simulink model "AC_motor_KDB_Roto_Day_Quan"  (R2019a)
settings: Solver=VariableStepAuto  StartTime=0.0  StopTime=10.0  RelTol=1e-3
libraries: powerlib x13
settings Model: Creator=Admin  LastModifiedBy=Admin

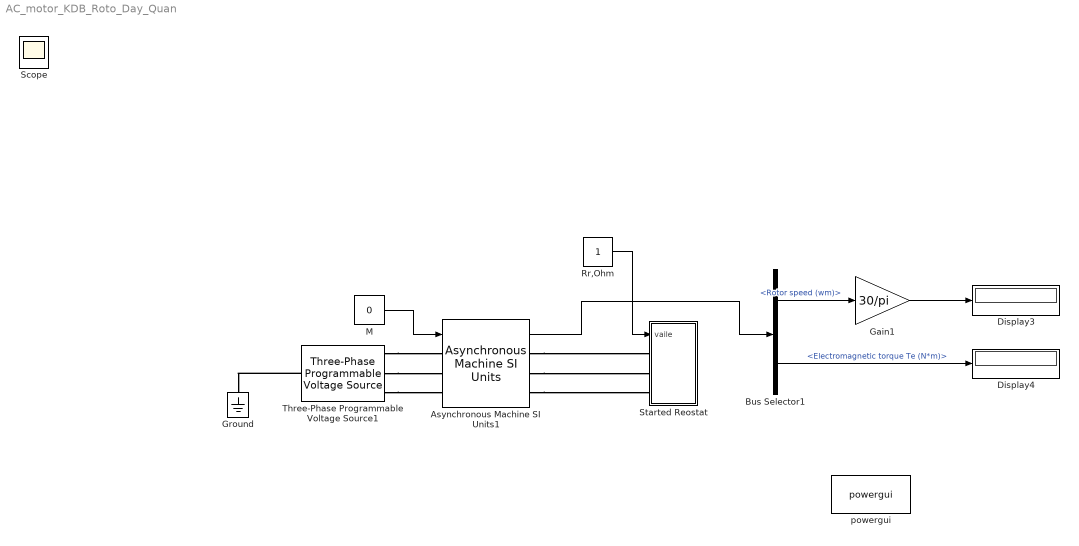
== system AC_motor_KDB_Roto_Day_Quan ==
  Asynchronous Machine SI Units1 : powerlib/Machines/Asynchronous Machine SI Units  RotorType=Wound  PresetModel="15:  5.4 HP (4KW)   400 V  50Hz 1430 RPM"  MechanicalLoad=Torque Tm  ShowDetailedParameters=on  ReferenceFrame=Stationary  Units=SI  MeasurementBus=off  NominalParameters=[1000 380 50]  Stator=[3.28 0.0039]  Rotor=[1.167 0.0039]  Cage1=[0.4155 0.002066]  Cage2=[0.4168 0.0003495]  Lm=0.1671  Mechanical="[0.0058  0 2]"  PolePairs=2  InitialConditions=[0 0 0 0 0 0 0 0]  SimulateSaturation=off  Saturation=[14.03593122, 27.81365428, 53.79336849, 72.68890987, 97.98006896, 148.6815601, 215.7428561, 302.9841135, 428.7778367 ; 230, 322, 414, 460, 506, 552, 598, 644, 690]  LoadFlowParameters=1492000  TsPowergui=0  TsBlock=-1  IterativeModel=Trapezoidal non iterative  IterativeDiscreteModel=Trapezoidal non iterative  Pmec=1.492e+006
      settings: SourceProductName=Simscape Electrical
  Bus Selector1 : BusSelector  OutputSignals=Mechanical.Rotor speed (wm),Mechanical.Electromagnetic torque Te (N*m)
  Display3 : Display
  Display4 : Display
  Gain1 : Gain  Gain=30/pi
  Ground : powerlib/Elements/Ground  LConnTagsString=a
      settings: SourceProductName=Simscape Electrical
  M : Constant  Value=0
  Rr,Ohm : Constant
  Scope : Scope
  Started Reostat : Subsystem
  Three-Phase Programmable Voltage Source1 : powerlib/Electrical Sources/Three-Phase Programmable Voltage Source  PositiveSequence="[380  0 50]"  VariationEntity=None  VariationType=Table of time-amplitude pairs  VariationTypeAlt=Step  VariationStep=0.5  VariationRate=10  VariationMagnitude=0.3  VariationFrequency=2  VariationTiming=[1 2]  VariationPhaseA=off  Amplitudes=[1 0.8 1.2 1.0]  TimeValues=[0 0.1 0.15 0.2]  HarmonicGeneration=off  HarmonicA=[3 0.2 -25 0]  HarmonicB=[2 0.15 35 2]  Timing="[0.05  3]"  BusType=swing  Pref=0  Qref=0  Qmin=-inf  Qmax=inf
      settings: SourceProductName=Simscape Electrical
  powergui : powerlib/powergui  Priority=1  SimulationMode=Continuous  SampleTime=50e-6  frequency=60  Iterations=50  frequencyindice=50  Pbase=100e6  ErrMax=1e-4  UnitsV=kV  UnitsW=MW  buscounter=0  FunctionMessages=off  echomessages=off  EnableUseOfTLC=off  CurrentSourceSwitches=off  DisableSnubberDevices=off  DisableRonSwitches=off  DisableVfSwitches=off  DisplayEquations=off  AutomaticDiscreteSolvers=off  SolverType=Tustin/Backward Euler (TBE)  Interpol=off  ExternalGateDelay=off  methode=off  Ts=100  x0status=blocks  SPID=on  SwTol=0  HookPort=off  NonlinearTolerance=0  nMaxIteration=15  ContinueOnMaxIteration=off  RestoreLinks=warning  ResistiveCurrentMeasurement=off  Frange=[0:2:500]  Ylog=off  Xlog=on  ShowGrid=off  save=off  variable=ZData  structure=0  ZoomFFT=off  StartTime=0.0  cycles=1  DisplayStyle=1  fundamental=60  FreqAxis=off  MaxFrequency=1000  frequencyindicesteady=1  RmsSteady=1  display=off
      settings: SourceProductName=Simscape Electrical
  wires:
  Asynchronous Machine SI Units1/1 -> Bus Selector1/1
  Bus Selector1/1 -> Gain1/1  "<Rotor speed (wm)>"
  Gain1/1 -> Display3/1
  Bus Selector1/2 -> Display4/1  "<Electromagnetic torque Te (N*m)>"
  M/1 -> Asynchronous Machine SI Units1/1
  Rr,Ohm/1 -> Started Reostat/1(vaile)
  connections:
  Three-Phase Programmable Voltage Source1/LConn1 -- Ground/LConn1
  Three-Phase Programmable Voltage Source1/RConn1 -- Asynchronous Machine SI Units1/LConn1
  Three-Phase Programmable Voltage Source1/RConn2 -- Asynchronous Machine SI Units1/LConn2
  Three-Phase Programmable Voltage Source1/RConn3 -- Asynchronous Machine SI Units1/LConn3
  Asynchronous Machine SI Units1/RConn3 -- Started Reostat/LConn3
  Asynchronous Machine SI Units1/RConn2 -- Started Reostat/LConn2
  Asynchronous Machine SI Units1/RConn1 -- Started Reostat/LConn1

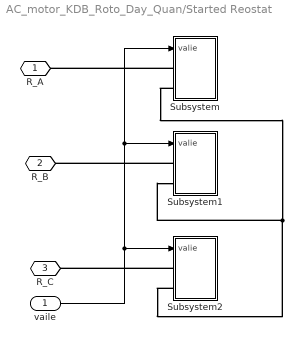
== system AC_motor_KDB_Roto_Day_Quan/Started Reostat ==
  vaile : Inport
  Subsystem : Subsystem
  Subsystem1 : Subsystem
  Subsystem2 : Subsystem
  R_A : PMIOPort  Side=Left
  R_B : PMIOPort  Port=2  Side=Left
  R_C : PMIOPort  Port=3  Side=Left
  wires:
  vaile/1 -> Subsystem2/1(valie), Subsystem1/1(valie), Subsystem/1(valie)
  connections:
  Subsystem/LConn1 -- R_A/RConn1
  Subsystem/LConn2 -- Subsystem2/LConn2 -- Subsystem1/LConn2
  Subsystem2/LConn1 -- R_C/RConn1
  Subsystem1/LConn1 -- R_B/RConn1

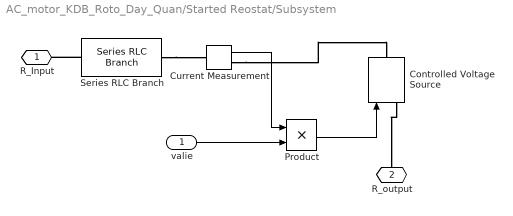
== system AC_motor_KDB_Roto_Day_Quan/Started Reostat/Subsystem ==
  valie : Inport
  Controlled Voltage Source : powerlib/Electrical Sources/Controlled Voltage Source  Initialize=on  Source_Type=AC  Amplitude=0  Phase=0  Frequency=0  Measurements=None
      settings: SourceProductName=Simscape Electrical
  Current Measurement : powerlib/Measurements/Current Measurement  PhasorSimulation=off  OutputType=Complex  PSBequivalent=0
      settings: SourceProductName=Simscape Electrical
  Product : Product
  Series RLC Branch : powerlib/Elements/Series RLC Branch  LConnTagsString=__new0  RConnTagsString=__new0  BranchType=R  Resistance=1  Inductance=1e-3  SetiL0=off  InitialCurrent=0  Capacitance=1e-6  Setx0=off  InitialVoltage=0  Measurements=None
      settings: SourceProductName=Simscape Electrical
  R_Input : PMIOPort  Side=Left
  R_output : PMIOPort  Port=2  Side=Left
  wires:
  Current Measurement/1 -> Product/1
  valie/1 -> Product/2
  Product/1 -> Controlled Voltage Source/1
  connections:
  Series RLC Branch/RConn1 -- Current Measurement/LConn1
  Current Measurement/RConn1 -- Controlled Voltage Source/RConn1
  Series RLC Branch/LConn1 -- R_Input/RConn1
  Controlled Voltage Source/LConn1 -- R_output/RConn1

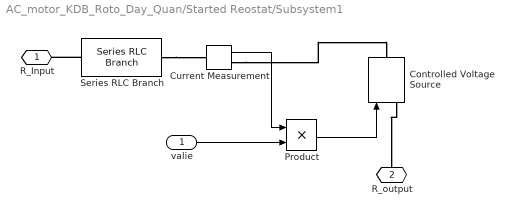
== system AC_motor_KDB_Roto_Day_Quan/Started Reostat/Subsystem1 ==
  valie : Inport
  Controlled Voltage Source : powerlib/Electrical Sources/Controlled Voltage Source  Initialize=on  Source_Type=AC  Amplitude=0  Phase=0  Frequency=0  Measurements=None
      settings: SourceProductName=Simscape Electrical
  Current Measurement : powerlib/Measurements/Current Measurement  PhasorSimulation=off  OutputType=Complex  PSBequivalent=0
      settings: SourceProductName=Simscape Electrical
  Product : Product
  Series RLC Branch : powerlib/Elements/Series RLC Branch  LConnTagsString=__new0  RConnTagsString=__new0  BranchType=R  Resistance=1  Inductance=1e-3  SetiL0=off  InitialCurrent=0  Capacitance=1e-6  Setx0=off  InitialVoltage=0  Measurements=None
      settings: SourceProductName=Simscape Electrical
  R_Input : PMIOPort  Side=Left
  R_output : PMIOPort  Port=2  Side=Left
  wires:
  Current Measurement/1 -> Product/1
  valie/1 -> Product/2
  Product/1 -> Controlled Voltage Source/1
  connections:
  Series RLC Branch/RConn1 -- Current Measurement/LConn1
  Current Measurement/RConn1 -- Controlled Voltage Source/RConn1
  Series RLC Branch/LConn1 -- R_Input/RConn1
  Controlled Voltage Source/LConn1 -- R_output/RConn1

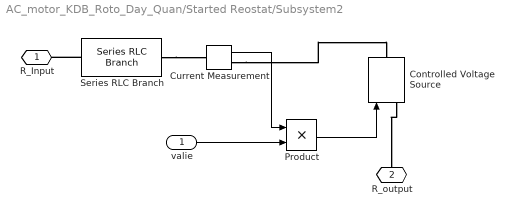
== system AC_motor_KDB_Roto_Day_Quan/Started Reostat/Subsystem2 ==
  valie : Inport
  Controlled Voltage Source : powerlib/Electrical Sources/Controlled Voltage Source  Initialize=on  Source_Type=AC  Amplitude=0  Phase=0  Frequency=0  Measurements=None
      settings: SourceProductName=Simscape Electrical
  Current Measurement : powerlib/Measurements/Current Measurement  PhasorSimulation=off  OutputType=Complex  PSBequivalent=0
      settings: SourceProductName=Simscape Electrical
  Product : Product
  Series RLC Branch : powerlib/Elements/Series RLC Branch  LConnTagsString=__new0  RConnTagsString=__new0  BranchType=R  Resistance=1  Inductance=1e-3  SetiL0=off  InitialCurrent=0  Capacitance=1e-6  Setx0=off  InitialVoltage=0  Measurements=None
      settings: SourceProductName=Simscape Electrical
  R_Input : PMIOPort  Side=Left
  R_output : PMIOPort  Port=2  Side=Left
  wires:
  Current Measurement/1 -> Product/1
  valie/1 -> Product/2
  Product/1 -> Controlled Voltage Source/1
  connections:
  Series RLC Branch/RConn1 -- Current Measurement/LConn1
  Current Measurement/RConn1 -- Controlled Voltage Source/RConn1
  Series RLC Branch/LConn1 -- R_Input/RConn1
  Controlled Voltage Source/LConn1 -- R_output/RConn1
